simulink model "gm_sampleModel1897_3_sub"  (R2023a)
settings: Solver=VariableStepAuto  StartTime=0.0  StopTime=10.0  RelTol=1e-3
libraries: simulink x2, hdlsllib x1
settings Model: Creator=user1  LastModifiedBy=user1
settings OptimizationCC: BlockReduction=off  ConditionallyExecuteInputs=off
settings DebuggingCC: InheritedTsInSrcMsg=none

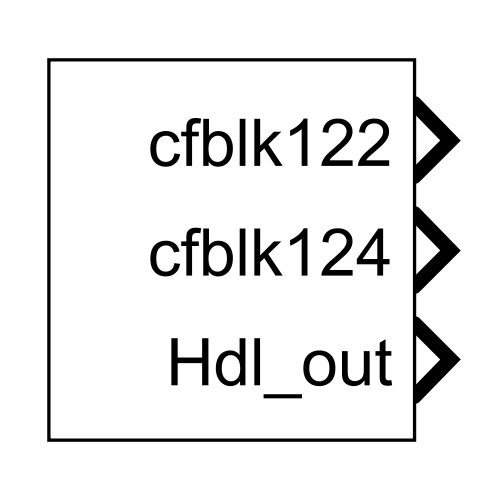
[thumbnail: Simulink's stored preview of the top-level diagram]
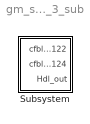
== system gm_sampleModel1897_3_sub ==
  Subsystem : Subsystem

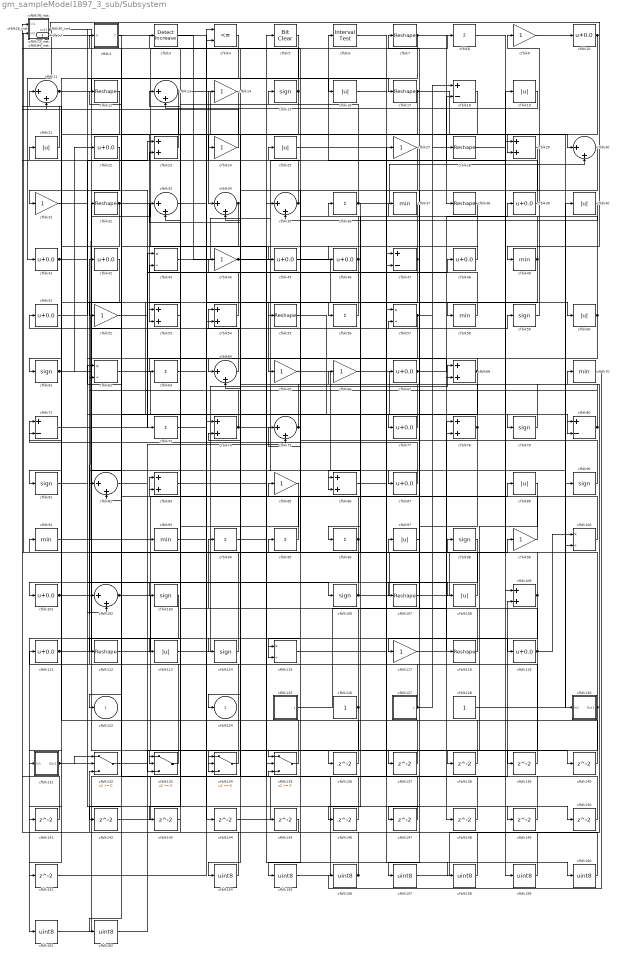
== system gm_sampleModel1897_3_sub/Subsystem ==
  cfblk{10,22,39,41..42,45..46,48,51,67,77,87,101,111,119} (15 alike) : Bias  Bias=0.0  SaturateOnIntegerOverflow=off
  cfblk{43,57,62,100,115} (5 alike) : Product  Inputs=*/  OutDataTypeStr=uint8  RndMeth=Zero  SaturateOnIntegerOverflow=on
  cfblk{11,13,30,33..35,64,75,82,102} (10 alike) : Sum  Inputs=|++  OutDataTypeStr=uint8
  cfblk{15,59,61,79,81,90,98,103,106,114} (10 alike) : Signum
  cfblk104_inst : Subsystem
  cfblk105_inst : Subsystem
  cfblk{7,12,17,28,32,38,55,107,112,118} (10 alike) : Reshape
  cfblk{16,19,21,25,40,60,89,97,108,113} (10 alike) : Abs  OutDataTypeStr=uint8  SaturateOnIntegerOverflow=off
  cfblk{23,29,53..54,68,74,78,83,86,109} (10 alike) : Sum  OutDataTypeStr=uint8
  cfblk116_inst : Subsystem
  cfblk{9,14,24,27,31,44,52,65..66,85,99,117} (12 alike) : Gain  OutDataTypeStr=uint8
  cfblk125 : Subsystem  mask(Counter Limited){uplimit=double(7), tsamp=double(-1)}
      mask prompts: uplimit "Simulink:masks:UpperLimit_MP"; tsamp "Simulink:masks:SampleTime_MP"
      mask help: Simulink:masks:CounterLimited_MD
      mask init:
      | nbits = double(8);
      | tsamp = double(-1);
      | uplimit = double(7);
  cfblk126 : Constant  OutDataTypeStr=uint8  SampleTime=-1
  cfblk127 : Subsystem  mask(Counter Free-Running){NumBits=double(16), tsamp=double(-1)}
      mask prompts: NumBits "Simulink:masks:NumberOfBits_MP"; tsamp "Simulink:masks:SampleTime_MP"
      mask help: Simulink:masks:CounterFreeRunning_MD
  cfblk128 : Constant  OutDataTypeStr=uint8  SampleTime=-1
  cfblk130 : Subsystem
  cfblk131 : Subsystem
  cfblk{132..135} (4 alike) : Switch  OutDataTypeStr=uint8  SaturateOnIntegerOverflow=off  InputSameDT=off
  cfblk{136..151} (16 alike) : Delay  SampleTime=1
  cfblk{154..162} (9 alike) : DataTypeConversion  OutDataTypeStr=uint8  SaturateOnIntegerOverflow=off  RndMeth=Floor
  cfblk{18,47,71,80} (4 alike) : Sum  Inputs=+-  OutDataTypeStr=uint8
  cfblk2 : Subsystem  mask(Detect Rise Nonnegative){vinit=double(0), InputProcessing=Elements as channels (sample based), OutDataTypeStr=uint8}
      mask prompts: vinit "Simulink:masks:InitialCondition_MP"; InputProcessing "Simulink:masks:InputProcessing_MP"; OutDataTypeStr "Simulink:masks:OutputDataType_MP"
      mask help: Simulink:masks:DetectRiseNonnegative_MD
      mask init:
      | InputProcessing = 'Elements as channels (sample based)';
      | OutDataTypeStr = 'uint8';
      | vinit = double(0);
      mask TypeOptions InputProcessing: Simulink:masks:ColumnsAsChannelsFrameBased | Simulink:masks:ElementsAsChannelsSampleBased
      mask TypeOptions OutDataTypeStr: Simulink:masks:uint8 | Simulink:masks:boolean
      mask Display: fprintf('U >= 0\n&  NOT\nU/z >= 0')
  cfblk26_inst : Subsystem
  cfblk3 : simulink/Logic and Bit Operations/Detect Increase  vinit=0.0  OutDataTypeStr=uint8
      settings: LibrarySourceBlock=|
      | hdlsllib/Logic and Bit
      | Operations/Detect
      | Increase
  cfblk{8,36,56,63,73,94..96} (8 alike) : Sum  Inputs=+  OutDataTypeStr=uint8
  cfblk{37,49,58,70,91,93} (6 alike) : MinMax  OutDataTypeStr=uint8
  cfblk4 : RelationalOperator  Operator=<=  OutDataTypeStr=boolean  InputSameDT=off
  cfblk5 : simulink/Logic and Bit Operations/Bit Clear  iBit=0
      settings: LibrarySourceBlock=|
      | hdlsllib/Logic and Bit
      | Operations/Bit Clear
  cfblk50_inst : Subsystem
  cfblk6 : hdlsllib/Logic and Bit Operations/Interval Test  IntervalClosedRight=on  uplimit=0.5  IntervalClosedLeft=on  lowlimit=-0.5  OutDataTypeStr=uint8
  cfblk72_inst : Subsystem
  cfblk76_inst : Subsystem
  cfblk84_inst : Subsystem
  cfblk122 : Outport  OutDataTypeStr=uint8  SampleTime=1  VectorParamsAs1DForOutWhenUnconnected=off
  cfblk124 : Outport  Port=2  OutDataTypeStr=uint8  SampleTime=1  VectorParamsAs1DForOutWhenUnconnected=off
  Hdl_out : Outport  Port=3  OutDataTypeStr=uint8  SampleTime=1
  wires:
  cfblk10/1 -> cfblk53/2, cfblk34/1
  cfblk100/1 -> cfblk51/1
  cfblk101/1 -> cfblk97/1, cfblk99/1
  cfblk102/1 -> cfblk137/1, cfblk136/1
  cfblk103/1 -> cfblk161/1
  cfblk104_inst/1(out1) -> cfblk79/1
  cfblk105_inst/1(out1) -> cfblk56/1
  cfblk106/1 -> cfblk98/1, cfblk72_inst/2(in2)
  cfblk107/1 -> cfblk19/1
  cfblk108/1 -> cfblk21/1
  cfblk109/1 -> cfblk135/3, cfblk36/1
  cfblk11/1 -> cfblk29/2, cfblk17/1, cfblk133/2
  cfblk111/1 -> cfblk32/1, cfblk8/1
  cfblk112/1 -> cfblk85/1
  cfblk113/1 -> cfblk68/1
  cfblk114/1 -> cfblk105_inst/1(in1)
  cfblk115/1 -> cfblk47/2
  cfblk116_inst/1(out1) -> cfblk49/1, cfblk73/1
  cfblk117/1 -> cfblk78/1
  cfblk118/1 -> cfblk43/2
  cfblk119/1 -> cfblk7/1, cfblk134/3, cfblk100/1
  cfblk12/1 -> cfblk81/1
  cfblk125/1(y) -> cfblk78/2
  cfblk126/1 -> cfblk133/3, cfblk94/1
  cfblk127/1(y) -> cfblk42/1, cfblk28/1, cfblk157/1
  cfblk128/1 -> cfblk40/1
  cfblk13/1 -> cfblk30/1, cfblk112/1
  cfblk130/1(Out1) -> cfblk25/1, cfblk134/2
  cfblk131/1(Out1) -> cfblk132/2, cfblk132/1
  cfblk132/1 -> cfblk95/1
  cfblk133/1 -> cfblk12/1
  cfblk134/1 -> cfblk111/1
  cfblk135/1 -> cfblk91/1
  cfblk136/1 -> cfblk71/1
  cfblk137/1 -> cfblk74/2
  cfblk138/1 -> cfblk11/1
  cfblk139/1 -> cfblk54/1
  cfblk14/1 -> cfblk53/1
  cfblk140/1 -> cfblk47/1
  cfblk141/1 -> cfblk116_inst/1(in1)
  cfblk142/1 -> cfblk57/1
  cfblk143/1 -> cfblk13/1
  cfblk144/1 -> cfblk109/2
  cfblk145/1 -> cfblk132/3
  cfblk146/1 -> cfblk64/2
  cfblk147/1 -> cfblk2/1(U)
  cfblk148/1 -> cfblk82/2
  cfblk149/1 -> cfblk23/2
  cfblk15/1 -> cfblk50_inst/1(in1), cfblk134/1
  cfblk150/1 -> cfblk135/2
  cfblk151/1 -> cfblk4/2
  cfblk154/1 -> cfblk76_inst/1(in1)
  cfblk155/1 -> cfblk27/1
  cfblk156/1 -> cfblk84_inst/2(in2), cfblk76_inst/2(in2)
  cfblk157/1 -> cfblk70/1
  cfblk158/1 -> cfblk84_inst/1(in1)
  cfblk159/1 -> cfblk83/1
  cfblk16/1 -> cfblk139/1
  cfblk160/1 -> cfblk83/2
  cfblk161/1 -> cfblk5/1
  cfblk162/1 -> cfblk93/1
  cfblk17/1 -> cfblk103/1, cfblk100/2
  cfblk18/1 -> cfblk124/1
  cfblk19/1 -> cfblk13/2
  cfblk2/1(Y) -> cfblk52/1
  cfblk21/1 -> cfblk104_inst/1(in1)
  cfblk22/1 -> cfblk31/1
  cfblk23/1 -> cfblk116_inst/2(in2)
  cfblk24/1 -> cfblk11/2
  cfblk25/1 -> cfblk108/1
  cfblk26_inst/1(out1) -> cfblk119/1
  cfblk27/1 -> cfblk154/1
  cfblk28/1 -> cfblk159/1
  cfblk29/1 -> cfblk117/1
  cfblk3/1 -> cfblk74/1
  cfblk30/1 -> cfblk115/2
  cfblk31/1 -> cfblk114/1
  cfblk32/1 -> cfblk61/1, cfblk145/1
  cfblk33/1 -> cfblk150/1
  cfblk34/1 -> cfblk133/1, cfblk142/1
  cfblk35/1 -> cfblk26_inst/1(in1), cfblk14/1
  cfblk36/1 -> cfblk30/2, cfblk26_inst/2(in2), cfblk96/1
  cfblk37/1 -> cfblk102/1
  cfblk38/1 -> cfblk115/1
  cfblk39/1 -> cfblk6/1
  cfblk4/1 -> cfblk82/1
  cfblk40/1 -> cfblk35/2
  cfblk41/1 -> cfblk68/2, cfblk106/1
  cfblk42/1 -> cfblk101/1
  cfblk43/1 -> cfblk18/2
  cfblk44/1 -> cfblk29/1, cfblk148/1
  cfblk45/1 -> cfblk90/1
  cfblk46/1 -> cfblk54/2, cfblk105_inst/2(in2), Hdl_out/1
  cfblk47/1 -> cfblk86/2, cfblk45/1, cfblk65/1
  cfblk48/1 -> cfblk46/1
  cfblk49/1 -> cfblk107/1, cfblk104_inst/2(in2)
  cfblk5/1 -> cfblk162/1
  cfblk50_inst/1(out1) -> cfblk41/1
  cfblk51/1 -> cfblk23/1
  cfblk52/1 -> cfblk57/2
  cfblk53/1 -> cfblk143/1
  cfblk54/1 -> cfblk3/1
  cfblk55/1 -> cfblk80/2
  cfblk56/1 -> cfblk55/1
  cfblk57/1 -> cfblk64/1, cfblk18/1
  cfblk58/1 -> cfblk44/1
  cfblk59/1 -> cfblk9/1
  cfblk6/1 -> cfblk160/1
  cfblk60/1 -> cfblk50_inst/2(in2), cfblk146/1
  cfblk61/1 -> cfblk59/1, cfblk22/1, cfblk144/1
  cfblk62/1 -> cfblk118/1
  cfblk63/1 -> cfblk86/1
  cfblk64/1 -> cfblk4/1
  cfblk65/1 -> cfblk130/1(In1)
  cfblk66/1 -> cfblk80/1
  cfblk67/1 -> cfblk39/1, cfblk140/1
  cfblk68/1 -> cfblk122/1, cfblk63/1
  cfblk7/1 -> cfblk38/1, cfblk151/1
  cfblk70/1 -> cfblk156/1
  cfblk71/1 -> cfblk48/1
  cfblk72_inst/1(out1) -> cfblk77/1
  cfblk73/1 -> cfblk135/1
  cfblk74/1 -> cfblk33/2, cfblk109/1
  cfblk75/1 -> cfblk33/1, cfblk155/1
  cfblk76_inst/1(out1) -> cfblk149/1, cfblk58/1
  cfblk77/1 -> cfblk43/1
  cfblk78/1 -> cfblk34/2, cfblk147/1
  cfblk79/1 -> cfblk66/1
  cfblk8/1 -> cfblk60/1
  cfblk80/1 -> cfblk72_inst/1(in1), cfblk62/2
  cfblk81/1 -> cfblk102/2
  cfblk82/1 -> cfblk87/1
  cfblk83/1 -> cfblk158/1
  cfblk84_inst/1(out1) -> cfblk16/1
  cfblk85/1 -> cfblk113/1
  cfblk86/1 -> cfblk67/1
  cfblk87/1 -> cfblk71/2
  cfblk89/1 -> cfblk138/1
  cfblk9/1 -> cfblk10/1
  cfblk90/1 -> cfblk15/1
  cfblk91/1 -> cfblk75/2
  cfblk93/1 -> cfblk89/1
  cfblk94/1 -> cfblk35/1
  cfblk95/1 -> cfblk24/1
  cfblk96/1 -> cfblk62/1, cfblk131/1(In1)
  cfblk97/1 -> cfblk37/1
  cfblk98/1 -> cfblk141/1
  cfblk99/1 -> cfblk75/1

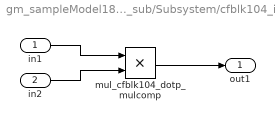
== system gm_sampleModel1897_3_sub/Subsystem/cfblk104_inst ==
  in1 : Inport  OutDataTypeStr=uint8  SampleTime=1
  in2 : Inport  Port=2  OutDataTypeStr=uint8  SampleTime=1
  mul_cfblk104_dotp_mulcomp : Product  Inputs=**  OutDataTypeStr=uint8  SampleTime=1
  out1 : Outport  OutDataTypeStr=uint8  SampleTime=1
  wires:
  in1/1 -> mul_cfblk104_dotp_mulcomp/1
  in2/1 -> mul_cfblk104_dotp_mulcomp/2
  mul_cfblk104_dotp_mulcomp/1 -> out1/1

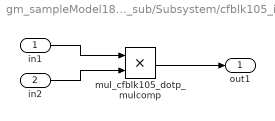
== system gm_sampleModel1897_3_sub/Subsystem/cfblk105_inst ==
  in1 : Inport  OutDataTypeStr=uint8  SampleTime=1
  in2 : Inport  Port=2  OutDataTypeStr=uint8  SampleTime=1
  mul_cfblk105_dotp_mulcomp : Product  Inputs=**  OutDataTypeStr=uint8  SampleTime=1
  out1 : Outport  OutDataTypeStr=uint8  SampleTime=1
  wires:
  in1/1 -> mul_cfblk105_dotp_mulcomp/1
  in2/1 -> mul_cfblk105_dotp_mulcomp/2
  mul_cfblk105_dotp_mulcomp/1 -> out1/1

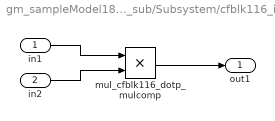
== system gm_sampleModel1897_3_sub/Subsystem/cfblk116_inst ==
  in1 : Inport  OutDataTypeStr=uint8  SampleTime=1
  in2 : Inport  Port=2  OutDataTypeStr=uint8  SampleTime=1
  mul_cfblk116_dotp_mulcomp : Product  Inputs=**  OutDataTypeStr=uint8  SampleTime=1
  out1 : Outport  OutDataTypeStr=uint8  SampleTime=1
  wires:
  in1/1 -> mul_cfblk116_dotp_mulcomp/1
  in2/1 -> mul_cfblk116_dotp_mulcomp/2
  mul_cfblk116_dotp_mulcomp/1 -> out1/1

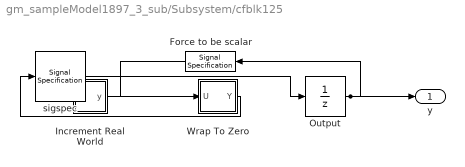
== system gm_sampleModel1897_3_sub/Subsystem/cfblk125 ==
  Force to be scalar : SignalSpecification  DisableCoverage=on  Dimensions=1
  Increment Real World : Subsystem  mask(Real World Value Increment){}
      mask help: Simulink:masks:RealWorldValueIncrement_MD
      mask Display: disp('V++')
  Output : UnitDelay  InitialCondition=0.0  SampleTime=tsamp  HasFrameUpgradeWarning=on
  Wrap To Zero : Subsystem  mask(Wrap To Zero){Threshold=double(7)}
      mask prompts: Threshold "Simulink:masks:Threshold_MP"
      mask help: Simulink:masks:WrapToZero_MD
  sigspec : SignalSpecification  OutDataTypeStr=uint8  Dimensions=1
  y : Outport  SampleTime=1
  wires:
  Force to be scalar/1 -> Increment Real World/1(u)
  Increment Real World/1(y) -> Wrap To Zero/1(U)
  Output/1 -> Force to be scalar/1, y/1
  Wrap To Zero/1(Y) -> sigspec/1
  sigspec/1 -> Output/1

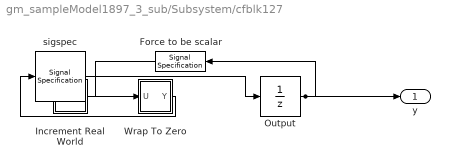
== system gm_sampleModel1897_3_sub/Subsystem/cfblk127 ==
  Force to be scalar : SignalSpecification  DisableCoverage=on  Dimensions=1
  Increment Real World : Subsystem  mask(Real World Value Increment){}
      mask help: Simulink:masks:RealWorldValueIncrement_MD
      mask Display: disp('V++')
  Output : UnitDelay  InitialCondition=0.0  SampleTime=tsamp  HasFrameUpgradeWarning=on
  Wrap To Zero : Subsystem  mask(Wrap To Zero){Threshold=double(65535)}
      mask prompts: Threshold "Simulink:masks:Threshold_MP"
      mask help: Simulink:masks:WrapToZero_MD
  sigspec : SignalSpecification  OutDataTypeStr=uint16  Dimensions=1
  y : Outport  SampleTime=1
  wires:
  Force to be scalar/1 -> Increment Real World/1(u)
  Increment Real World/1(y) -> Wrap To Zero/1(U)
  Output/1 -> Force to be scalar/1, y/1
  Wrap To Zero/1(Y) -> sigspec/1
  sigspec/1 -> Output/1

== system gm_sampleModel1897_3_sub/Subsystem/cfblk130 ==
  In1 : Inport  OutDataTypeStr=uint8  PortDimensions=1  SampleTime=1
  Out1 : Outport  SampleTime=1
  wires:
  In1/1 -> Out1/1

== system gm_sampleModel1897_3_sub/Subsystem/cfblk131 ==
  In1 : Inport  OutDataTypeStr=uint8  PortDimensions=1  SampleTime=1
  Out1 : Outport  SampleTime=1
  wires:
  In1/1 -> Out1/1

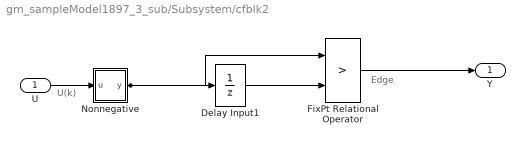
== system gm_sampleModel1897_3_sub/Subsystem/cfblk2 ==
  note: U(k)
  note: Edge
  U : Inport  OutDataTypeStr=uint8  SampleTime=1
  Delay Input1 : UnitDelay  Description=Store in Global RAM  DisableCoverage=on  InitialCondition=vinit  SampleTime=-1  HasFrameUpgradeWarning=on
  FixPt Relational Operator : RelationalOperator  Operator=>  OutDataTypeStr=fixdt(0, 8)  ZeroCross=off  InputSameDT=off
  Nonnegative : Subsystem  mask(Compare To Zero){relop=>=, OutDataTypeStr=boolean, ZeroCross=off}
      mask prompts: relop "Simulink:masks:Operator_MP"; OutDataTypeStr "Simulink:masks:OutputDataType_MP"; ZeroCross "Simulink:masks:EnableZerocrossingDetection_MP"
      mask help: Simulink:masks:CompareToZero_MD
      mask init:
      | OutDataTypeStr = 'boolean';
      | ZeroCross = 'off';
      | blkName = 'sampleModel1897_3_sub/Subsystem/cfblk2/Nonnegative';
      | relop = '>=';
      | setValue = 'boolean';
      mask TypeOptions relop: == | ~= | < | <= | >= | >
      mask TypeOptions OutDataTypeStr: Simulink:masks:uint8 | Simulink:masks:boolean
      mask Callback ZeroCross: sl('zeroCrossEnable', gcbh);
      mask Display: disp([relop,' 0'])
  Y : Outport  SampleTime=1
  wires:
  U/1 -> Nonnegative/1(u)
  Delay Input1/1 -> FixPt Relational Operator/2
  FixPt Relational Operator/1 -> Y/1
  Nonnegative/1(y) -> FixPt Relational Operator/1, Delay Input1/1

== system gm_sampleModel1897_3_sub/Subsystem/cfblk26_inst ==
  in1 : Inport  OutDataTypeStr=uint8  SampleTime=1
  in2 : Inport  Port=2  OutDataTypeStr=uint8  SampleTime=1
  mul_cfblk26_dotp_mulcomp : Product  Inputs=**  OutDataTypeStr=uint8  SampleTime=1
  out1 : Outport  OutDataTypeStr=uint8  SampleTime=1
  wires:
  in1/1 -> mul_cfblk26_dotp_mulcomp/1
  in2/1 -> mul_cfblk26_dotp_mulcomp/2
  mul_cfblk26_dotp_mulcomp/1 -> out1/1

== system gm_sampleModel1897_3_sub/Subsystem/cfblk50_inst ==
  in1 : Inport  OutDataTypeStr=uint8  SampleTime=1
  in2 : Inport  Port=2  OutDataTypeStr=uint8  SampleTime=1
  mul_cfblk50_dotp_mulcomp : Product  Inputs=**  OutDataTypeStr=uint8  SampleTime=1
  out1 : Outport  OutDataTypeStr=uint8  SampleTime=1
  wires:
  in1/1 -> mul_cfblk50_dotp_mulcomp/1
  in2/1 -> mul_cfblk50_dotp_mulcomp/2
  mul_cfblk50_dotp_mulcomp/1 -> out1/1

== system gm_sampleModel1897_3_sub/Subsystem/cfblk72_inst ==
  in1 : Inport  OutDataTypeStr=uint8  SampleTime=1
  in2 : Inport  Port=2  OutDataTypeStr=uint8  SampleTime=1
  mul_cfblk72_dotp_mulcomp : Product  Inputs=**  OutDataTypeStr=uint8  SampleTime=1
  out1 : Outport  OutDataTypeStr=uint8  SampleTime=1
  wires:
  in1/1 -> mul_cfblk72_dotp_mulcomp/1
  in2/1 -> mul_cfblk72_dotp_mulcomp/2
  mul_cfblk72_dotp_mulcomp/1 -> out1/1

== system gm_sampleModel1897_3_sub/Subsystem/cfblk76_inst ==
  in1 : Inport  OutDataTypeStr=uint8  SampleTime=1
  in2 : Inport  Port=2  OutDataTypeStr=uint8  SampleTime=1
  mul_cfblk76_dotp_mulcomp : Product  Inputs=**  OutDataTypeStr=uint8  SampleTime=1
  out1 : Outport  OutDataTypeStr=uint8  SampleTime=1
  wires:
  in1/1 -> mul_cfblk76_dotp_mulcomp/1
  in2/1 -> mul_cfblk76_dotp_mulcomp/2
  mul_cfblk76_dotp_mulcomp/1 -> out1/1

== system gm_sampleModel1897_3_sub/Subsystem/cfblk84_inst ==
  in1 : Inport  OutDataTypeStr=uint8  SampleTime=1
  in2 : Inport  Port=2  OutDataTypeStr=uint8  SampleTime=1
  mul_cfblk84_dotp_mulcomp : Product  Inputs=**  OutDataTypeStr=uint8  SampleTime=1
  out1 : Outport  OutDataTypeStr=uint8  SampleTime=1
  wires:
  in1/1 -> mul_cfblk84_dotp_mulcomp/1
  in2/1 -> mul_cfblk84_dotp_mulcomp/2
  mul_cfblk84_dotp_mulcomp/1 -> out1/1

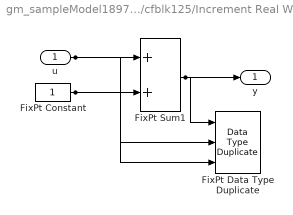
== system gm_sampleModel1897_3_sub/Subsystem/cfblk125/Increment Real World ==
  u : Inport  OutDataTypeStr=uint8  SampleTime=1
  FixPt Constant : Constant  DisableCoverage=on  OutDataTypeStr=Inherit: Inherit via back propagation  SampleTime=-1
  FixPt Data Type Duplicate : DataTypeDuplicate  DisableCoverage=on  NumInputPorts=3
  FixPt Sum1 : Sum  InputSameDT=on  OutDataTypeStr=Inherit: Inherit via back propagation  LockScale=on
  y : Outport  SampleTime=1
  wires:
  u/1 -> FixPt Sum1/1, FixPt Data Type Duplicate/2
  FixPt Constant/1 -> FixPt Sum1/2, FixPt Data Type Duplicate/3
  FixPt Sum1/1 -> FixPt Data Type Duplicate/1, y/1

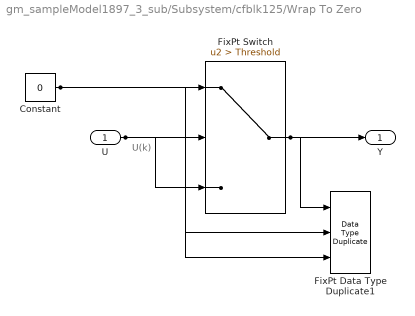
== system gm_sampleModel1897_3_sub/Subsystem/cfblk125/Wrap To Zero ==
  note: U(k)
  U : Inport  OutDataTypeStr=uint8  SampleTime=1
  Constant : Constant  DisableCoverage=on  Value=0  OutDataTypeStr=Inherit: Inherit via back propagation  SampleTime=-1
  FixPt Data Type Duplicate1 : DataTypeDuplicate  DisableCoverage=on  NumInputPorts=3
  FixPt Switch : Switch  Criteria=u2 > Threshold  Threshold=Threshold  OutDataTypeStr=Inherit: Inherit via back propagation  ZeroCross=off  SaturateOnIntegerOverflow=off  InputSameDT=off
  Y : Outport  SampleTime=1
  wires:
  U/1 -> FixPt Switch/3, FixPt Switch/2, FixPt Data Type Duplicate1/2
  Constant/1 -> FixPt Switch/1, FixPt Data Type Duplicate1/3
  FixPt Switch/1 -> FixPt Data Type Duplicate1/1, Y/1

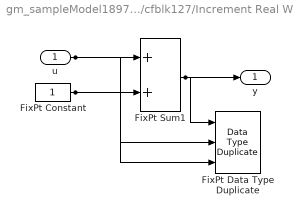
== system gm_sampleModel1897_3_sub/Subsystem/cfblk127/Increment Real World ==
  u : Inport  OutDataTypeStr=uint16  SampleTime=1
  FixPt Constant : Constant  DisableCoverage=on  OutDataTypeStr=Inherit: Inherit via back propagation  SampleTime=-1
  FixPt Data Type Duplicate : DataTypeDuplicate  DisableCoverage=on  NumInputPorts=3
  FixPt Sum1 : Sum  InputSameDT=on  OutDataTypeStr=Inherit: Inherit via back propagation  LockScale=on
  y : Outport  SampleTime=1
  wires:
  u/1 -> FixPt Sum1/1, FixPt Data Type Duplicate/2
  FixPt Constant/1 -> FixPt Sum1/2, FixPt Data Type Duplicate/3
  FixPt Sum1/1 -> FixPt Data Type Duplicate/1, y/1

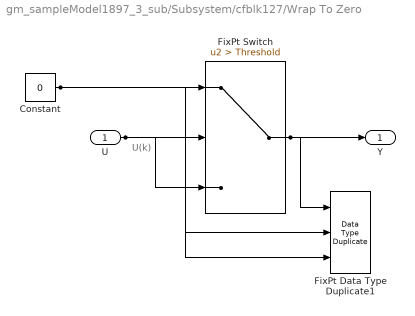
== system gm_sampleModel1897_3_sub/Subsystem/cfblk127/Wrap To Zero ==
  note: U(k)
  U : Inport  OutDataTypeStr=uint16  SampleTime=1
  Constant : Constant  DisableCoverage=on  Value=0  OutDataTypeStr=Inherit: Inherit via back propagation  SampleTime=-1
  FixPt Data Type Duplicate1 : DataTypeDuplicate  DisableCoverage=on  NumInputPorts=3
  FixPt Switch : Switch  Criteria=u2 > Threshold  Threshold=Threshold  OutDataTypeStr=Inherit: Inherit via back propagation  ZeroCross=off  SaturateOnIntegerOverflow=off  InputSameDT=off
  Y : Outport  SampleTime=1
  wires:
  U/1 -> FixPt Switch/3, FixPt Switch/2, FixPt Data Type Duplicate1/2
  Constant/1 -> FixPt Switch/1, FixPt Data Type Duplicate1/3
  FixPt Switch/1 -> FixPt Data Type Duplicate1/1, Y/1

== system gm_sampleModel1897_3_sub/Subsystem/cfblk2/Nonnegative ==
  u : Inport  OutDataTypeStr=uint8  SampleTime=1
  Compare : RelationalOperator  OutDataTypeStr=boolean  ZeroCross=off
  Constant : Constant  DisableCoverage=on  Value=0  OutDataTypeStr=Inherit: Inherit via back propagation  SampleTime=-1  PreserveConstantTs=on
  y : Outport  SampleTime=1
  wires:
  u/1 -> Compare/1
  Compare/1 -> y/1
  Constant/1 -> Compare/2
